simulink model "dSPACE_SIMULINK_MCV_2X"  (Simulink 7.6)
settings: Solver=ode1  StartTime=0.0  StopTime=Inf  FixedStep=(1/10000)  RelTol=1e-3
PostLoadFcn:
  | , if any(exist('dsrtsu_mdlpostloadfcn', 'file') == [2, 3, 6]), try dsrtsu_mdlpostloadfcn('Execute', bdroot); catch fprintf('Error in PostLoadFcn (dsrtsu_mdlpostloadfcn) for model "%s":\n %s\n', bdroot, lasterr); end, end,
values from neighbouring files (symbols this model uses):
  Ap = [0              Cy           0          0 ... (first row only)    [LoadnCheckModel.m]
  Ayaw = [0            Cx        0           0 ... (first row only)    [LoadnCheckModel.m]
  Bp = [0 0 0 KsEL*CwEL/tausEL]'    [LoadnCheckModel.m]
  Byaw = [0     0    0   KsAZ*CwAZ/tausAZ]'    [LoadnCheckModel.m]
  Cp = [1 0 0 0]    [LoadnCheckModel.m]
  Cyaw = [1 0 0 0]    [LoadnCheckModel.m]
  Kpf = KalmanFilter(Ap,Bp,Cp,Dp,Gp,W,V)    [GLTS_2X_master.m]
  Kpmcv = MCVController(Ap,Bp,Cp,Dp,Gp,W,gamma)    [GLTS_2X_master.m]
  Kyf = KalmanFilter(Ayaw, Byaw, Cyaw, Dyaw, Gyaw, W, V)    [GLTS_2X_master.m]
  Kymcv = MCVController(Ayaw,Byaw,Cyaw,Dyaw,Gyaw,W,gamma)    [GLTS_2X_master.m]
libraries: rtilib1104 x2, rti1104serlib x2, simulink x2
settings Model: DSRTSU_INTERNAL_RTI_VER=370  DSRTSU_INTERNAL_RTI_TYPE=rti1104  Creator=Team10  LastModifiedBy=Team10  TunableVars=Aye,Bye,Cye,Dye,Kpf,Kyf,Kyhat,Kylqg  TunableVarsStorageClass=Auto,Auto,Auto,Auto,Auto,Auto,Auto,Auto  TunableVarsTypeQualifier=,,,,,,,  BufferReuse=off
settings DataIOCC: LimitDataPoints=off
settings OptimizationCC: BlockReduction=off  ConditionallyExecuteInputs=off  OptimizeBlockIOStorage=off  BufferReuse=off  ExpressionFolding=off  LocalBlockOutputs=off
settings HardwareCC: ProdIntDivRoundTo=Zero  ProdEndianess=BigEndian  ProdHWDeviceType=Generic->Custom  TargetIntDivRoundTo=Zero  TargetEndianess=BigEndian  TargetHWDeviceType=Generic->Custom
settings RTWCC: SystemTargetFile=rti1104.tlc  MakeCommand=make_rti  TemplateMakefile=rti1104.tmf  Description=dSPACE DS1104 Hardware Platform  ProcessScript=rti1104_make_rtw_hook
settings STFCustomTargetCC: ParMdlRefBuildCompliant=on  GeneratePreprocessorConditionals=Disable all  SystemTargetFile=rti1104.tlc
settings GRTTargetCC: CompOptLevelCompliant=off  MatFileLogging=off  ExtModeMexFile=noextcomm
settings CustomProperty: DataType=RTWOptions_EnumType_C__dSPACE_matlab_rti1104_tlc_rti1104_1InitialSimState  Value=STOP
settings EnumStrPairs: String=RUN

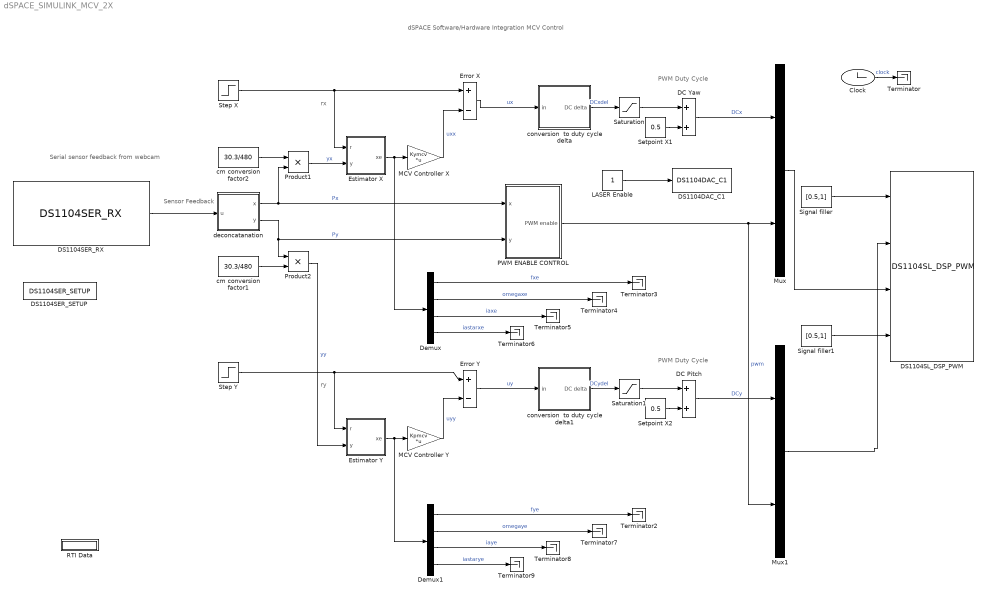
== system dSPACE_SIMULINK_MCV_2X ==
  note: rx
  note: PWM Duty Cycle
  note: dSPACE Software/Hardware Integration MCV Control
  note: Sensor Feedback
  note: Serial sensor feedback from webcam
  note: ry
  note: PWM Duty Cycle
  Clock : Clock
  DC Pitch : Sum
  DC Yaw : Sum
  DS1104DAC_C1 : rtilib1104/DS1104 MASTER PPC/DS1104DAC_C1  SystemSampleTime=-1  ChannelNo=1  InitValue=0  TermMode=0  TermValue=0  Reserved1=[]  Reserved2=[]  Reserved3=[]  Reserved4=[]  DialogFcn=gui1104dac  UnitName={ 'DS1104DAC_C'}  UnitValues={ 1 }  DSProperties=struct('RTI',struct('Version',uint32(1),'BlockType',struct('isSLSource',uint8(0),'isSLSink',uint8(1),'isHWSource',uint8(0),'isHWSink',uint8(1),'isSetup',uint8(0),'isInline',uint8(1),'isNonInline',uint8(0),'isInterrupt',uint8(0),'isChannelwise',uint8(1)),'IOBoardType','DS1104MASTER','UnitType','DAC','Identifier','DAC','DialogType','ML','BlockSet','NONE','SlaveProcessor','NONE'))
  DS1104SER_RX : rti1104serlib/DS1104SER_RX  SystemSampleTime=-1  Reserved1=[]  Reserved2=[]  Reserved3=[]  Reserved4=[]  DSProperties=struct('RTI',struct('IOBoardType',{{'DS1104','SER'}},'SlaveProcessor','NONE','Version',uint32(1),'BlockType',struct('isSLSource',uint8(1),'isSLSink',uint8(1),'isHWSource',uint8(0),'isHWSink',uint8(1),'isSetup',uint8(0),'isInline',uint8(1),'isNonInline',uint8(0),'isInterrupt',uint8(0),'isChannelwise',uint8(1)),'UnitType','GENSER','Identifier','RECEIVE','DialogType','ML','BlockSet','NONE'))  RTIBlockInterface=struct('BlockName',struct('Token',{{'DS1104SER_RX'}}),'InputPortsWidth',int32(1),'InputPortsActive',0,'InputPortsDataType',{{'SS_UINT32'}},'InputPortsName',{{'NumBytes'}},'OutputPortsWidth',int32([8 1 1]),'OutputPortsActive',[1 0 0],'OutputPortsDataType',{{'SS_UINT8','SS_UINT32','SS_INT32'}},'OutputPortsName',{{'RXBytes','NumRXBytes','Status'}},'BlockDisplay',{{['Serial Receive'],'center'}},'IconTransparency','on','ParameterTunableNames',{{}},'InitLevel',2,'DialogFcn','guigenserreceive','MaskDescription',['To read data from the UART SW FIFO.'])  RTIBlockParameters=struct('BoardNo',{{1,'ON',[1 1]}},'ChannelNo',{{1,'ON',[1 1]}},'ChannelNumOf',{{1,'OFF',[]}},'ReceptionDataMode',{{1,'OFF',[]}},'ParamTunableMode',{{2,'OFF',[]}},'BytesRefNumOfT',{{'1','OFF',[1 inf]}},'BytesRefNumOfNT',{{'8','OFF',[1 inf]}},'BytesRefNumOfMax',{{'1','OFF',[1 inf]}},'BytesRefNumOfMode',{{0,'OFF',[]}},'BytesActNumOfMode',{{0,'OFF',[]}},'ReceptionStatusMode',{{0,'OFF',[]}},'FifoSizeDefault',{{64,'OFF',[]}},'TLCFileName',{{'rtigenserreceive','OFF',[]}})  RTISFcnParameters=struct('BoardNo','double','ChannelNo','double','ChannelNumOf','double','ReceptionDataMode','double','ParamTunableMode','double','BytesRefNumOfT','double','BytesRefNumOfNT','double','BytesRefNumOfMax','double','BytesRefNumOfMode','double','BytesActNumOfMode','double','ReceptionStatusMode','double','TLCFileName','char')  RTIBlockParaDefault=struct('BoardNo',1,'ChannelNo',1,'ChannelNumOf',1,'ReceptionDataMode',1,'ParamTunableMode',1,'BytesRefNumOfT',1,'BytesRefNumOfNT',1,'BytesRefNumOfMax',1,'BytesRefNumOfMode',0,'BytesActNumOfMode',1,'ReceptionStatusMode',1,'FifoSizeDefault',64,'TLCFileName','rtigenserreceive')
  DS1104SER_SETUP : rti1104serlib/DS1104SER_SETUP  SystemSampleTime=-1  Reserved1=[]  Reserved2=[]  Reserved3=[]  Reserved4=[]  DSProperties=struct('RTI',struct('IOBoardType',{{'DS1104','SER'}},'SlaveProcessor','NONE','Version',uint32(2),'BlockType',struct('isSLSource',uint8(0),'isSLSink',uint8(0),'isHWSource',uint8(0),'isHWSink',uint8(0),'isSetup',uint8(1),'isInline',uint8(1),'isNonInline',uint8(0),'isInterrupt',uint8(0),'isChannelwise',uint8(1)),'UnitType','GENSER','Identifier','SETUP','DialogType','ML','BlockSet','NONE'))  RTIBlockInterface=struct('BlockName',struct('Token',{{'DS1104SER_SETUP'}}),'BlockDisplay',{{['Serial Setup'],'center'}},'IconTransparency','off','ParameterTunableNames',{{}},'InitLevel',1,'DialogFcn','guigensersetup','MaskDescription',['To set the global specifications for the UART interface.'])  RTIBlockParameters=struct('ParityMode',{{1,'OFF',[1 5]}},'TransceiverMode',{{1,'OFF',[]}},'QuartzFrequency',{{'16000000','OFF',[1 1]}},'BoardNo',{{1,'ON',[1 1]}},'ChannelNo',{{1,'ON',[1 1]}},'ChannelNumOf',{{1,'OFF',[]}},'BaudRate',{{'19200','OFF',[]}},'DataBitsNumOf',{{3,'OFF',[1 4]}},'StopBitsNumOf',{{1,'OFF',[1 3]}},'ReceiveIntLevelUart',{{3,'OFF',[1 4]}},'AutoflowMode',{{1,'OFF',[]}},'FifoSize',{{'64','OFF',[]}},'ReceiveIntLevelFifo',{{0,'OFF',[]}},'FifoOverrunMode',{{2,'OFF',[]}},'FifoBlockSize',{{'8','OFF',[]}},'TermMode',{{1,'OFF',[]}},'TLCFileName',{{'rtigensersetup','OFF',[]}})  RTISFcnParameters=struct('BoardNo','double','ChannelNo','double','ChannelNumOf','double','BaudRate','double','DataBitsNumOf','double','StopBitsNumOf','double','ParityMode','double','TransceiverMode','double','ReceiveIntLevelUart','double','AutoflowMode','double','FifoSize','double','ReceiveIntLevelFifo','double','FifoBlockSize','double','TermMode','double','QuartzFrequency','double','TLCFileName','char')  RTIBlockParaDefault=struct('ParityMode',1,'TransceiverMode',1,'QuartzFrequency',16000000,'BoardNo',1,'ChannelNo',1,'ChannelNumOf',1,'BaudRate',115200,'DataBitsNumOf',4,'StopBitsNumOf',1,'ReceiveIntLevelUart',4,'AutoflowMode',0,'FifoSize',64,'ReceiveIntLevelFifo',0,'FifoOverrunMode',1,'FifoBlockSize',0,'TermMode',1,'TLCFileName','rtigensersetup')
  DS1104SL_DSP_PWM : rtilib1104/DS1104 SLAVE DSP/DS1104SL_DSP_PWM  SystemSampleTime=-1  Parameters=[]  TDef=[]  BoardType=[]  PwmMode=[]  Frequency=[]  InitValue=[]  TermMode=[]  TermValue=[]  Polarity=[]  DialogFcn=[]  Reserved1=[]  Reserved2=[]  Reserved3=[]  Reserved4=[]  Revision=[]  UnitName=[]  UnitValues=[]  DSProperties=struct('RTI',struct('Version',uint32(2),'BlockType',struct('isSLSource',uint8(0),'isSLSink',uint8(1),'isHWSource',uint8(0),'isHWSink',uint8(1),'isSetup',uint8(0),'isInline',uint8(1),'isNonInline',uint8(0),'isInterrupt',uint8(0),'isChannelwise',uint8(0)),'IOBoardType','DS1104SLAVE','UnitType','PWM','Identifier','PWM','DialogType','ML','BlockSet','NONE','SlaveProcessor','F240'))  RTIBlockInterface=struct('InputPortsActive',[1 1 1 1],'InputPortsWidth',int32([2 2 2 2]),'InputPortsName',{{['PWM Channel 1'],['PWM Channel 2'],['PWM Channel 3'],['PWM Channel 4']}},'IWork',{{{'',uint32(4)}}},'DialogFcn','rti1104slavepwmgui','InitLevel',1,'BlockDisplay',{{'','auto'}},'IconTransparency','on','MultiSFcn',4,'BlockName',struct('Token',{{'DS1104SL_DSP_PWM'}}))  RTIBlockParameters=struct('PWMSymmetryMode',{{1,'OFF',[]}},'PWMFrequency',{{'100000','OFF',[]}},'PWMPolarityMode',{{[1 1 1 1 1],'OFF',[]}},'ChannelNo',{{[1 2 3 4],'OFF',[]}},'SuspendModeInit',{{[1 1 1 1 1],'OFF',[]}},'TTLModeInit',{{[2 2 2 2 2],'OFF',[]}},'DutyCycleInitValueCh1',{{'0.5','OFF',[]}},'DutyCycleInitValueCh2',{{'0.5','OFF',[]}},'DutyCycleInitValueCh3',{{'0.5','OFF',[]}},'DutyCycleInitValueCh4',{{'0.5','OFF',[]}},'DutyCycleInitValueCh5',{{'0.5','OFF',[]}},'EnablePWMStop',{{[1 1 1 1 0],'OFF',[]}},'SuspendModeTerm',{{[1 1 1 1 1],'OFF',[]}},'TTLModeTerm',{{[2 2 2 2 2],'OFF',[]}},'DutyCycleTermValueCh1',{{'0.5','OFF',[]}},'DutyCycleTermValueCh2',{{'0.5','OFF',[]}},'DutyCycleTermValueCh3',{{'0.5','OFF',[]}},'DutyCycleTermValueCh4',{{'0.5','OFF',[]}},'DutyCycleTermValueCh5',{{'0.5','OFF',[]}},'TLCFileName',{{'rti1104pwm','OFF',[]}})  RTISFcnParameters=struct('PWMSymmetryMode','double','PWMFrequency','double','PWMPolarityMode','double','ChannelNo','double','SuspendModeInit','double','TTLModeInit','double','DutyCycleInitValueCh1','double','DutyCycleInitValueCh2','double','DutyCycleInitValueCh3','double','DutyCycleInitValueCh4','double','EnablePWMStop','double','SuspendModeTerm','double','TTLModeTerm','double','DutyCycleTermValueCh1','double','DutyCycleTermValueCh2','double','DutyCycleTermValueCh3','double','DutyCycleTermValueCh4','double','TLCFileName','char')  RTIBlockParaDefault=struct('PWMSymmetryMode',1,'PWMFrequency',100,'PWMPolarityMode',[1 1 1 1 1],'ChannelNo',[1 2 3 4],'SuspendModeInit',[1 1 1 1 1],'TTLModeInit',[2 2 2 2 2],'DutyCycleInitValueCh1',0.5,'DutyCycleInitValueCh2',0.5,'DutyCycleInitValueCh3',0.5,'DutyCycleInitValueCh4',0.5,'DutyCycleInitValueCh5',0.5,'EnablePWMStop',[1 1 1 1 0],'SuspendModeTerm',[1 1 1 1 1],'TTLModeTerm',[2 2 2 2 2],'DutyCycleTermValueCh1',0.5,'DutyCycleTermValueCh2',0.5,'DutyCycleTermValueCh3',0.5,'DutyCycleTermValueCh4',0.5,'DutyCycleTermValueCh5',0.5,'TLCFileName','rti1104pwm')
  Demux : Demux
  Demux1 : Demux
  Error X : Sum  Inputs=+-
  Error Y : Sum  Inputs=+-
  Estimator X : Subsystem
  Estimator Y : Subsystem
  LASER Enable : Constant
  MCV Controller X : Gain  Gain=Kymcv  Multiplication=Matrix(K*u)
  MCV Controller Y : Gain  Gain=Kpmcv  Multiplication=Matrix(K*u)
  Mux : Mux  Inputs=2
  Mux1 : Mux  Inputs=2
  PWM ENABLE CONTROL : Subsystem
  Product1 : Product  RndMeth=Zero
  Product2 : Product  RndMeth=Zero
  RTI Data : Subsystem  Tag=struct('RTIDataServer',struct('RTIDataServerVs','2','RTIModelDescription','struct(''main'',''dSPACE_SIMULINK_MCV_2X'',''sub'','''',''isMp'',0)'))  LoadFcn="if exist('rtidc'), try,  rtidc('DataHostBlockClbLoad', gcbh); catch, disp(['Warning: ''LoadFcn'' for RTI Data block failed: ' lasterr]); end, end,"
      settings: CopyFcn="if exist('rtidc'), try,  rtidc('DataHostBlockClbCopy', gcbh); catch, disp(['Warning: ''CopyFcn'' for RTI Data block failed: ' lasterr]); end, end,"  DeleteFcn="if exist('rtidc'), try,  rtidc('DataHostBlockClbDelete', gcbh); catch, disp(['Warning: ''DeleteFcn'' for RTI Data block failed: ' lasterr]); end, end,"  ModelCloseFcn="if exist('rtidc'), try,  rtidc('DataHostBlockClbModelClose', gcbh); catch, disp(['Warning: ''ModelCloseFcn'' for RTI Data block failed: ' lasterr]); end, end,"  PreSaveFcn="if exist('rtidc'), try,  rtidc('DataHostBlockClbPreSave', gcbh); catch, disp(['Warning: ''PreSaveFcn'' for RTI Data block failed: ' lasterr]); end, end,"  PostSaveFcn="if exist('rtidc'), try,  rtidc('DataHostBlockClbPostSave', gcbh); catch, disp(['Warning: ''PostSaveFcn'' for RTI Data block failed: ' lasterr]); end, end,"  NameChangeFcn="if exist('rtidc'), try,  rtidc('DataHostBlockClbNameChange', gcbh); catch, disp(['Warning: ''NameChangeFcn'' for RTI Data block failed: ' lasterr]); end, end,"
      mask Type: RTI_DATA_HOST
      mask Description:
      | RTI Data Block.
      | This block is used by RTI to store internal model-dependent data.
      | Please keep this block on the root level of the model. Deleting this block will result in data loss.
      | 
      | NEVER DELETE OR COPY THIS BLOCK!
      mask Help:
      | RTI Data Block.
      | This block is used by RTI to store internal model-dependent data.
      | Please keep this block on the root level of the model. Deleting this block will result in data loss.
      | 
      | NEVER DELETE OR COPY THIS BLOCK!
      mask Display:
      | text(0.5, 0.5, 'RTI Data', 'HorizontalAlignment', 'center');
      | plot([1 0]);
  Saturation : Saturate
  Saturation1 : Saturate
  Setpoint X1 : Constant  Value=0.5
  Setpoint X2 : Constant  Value=0.5
  Signal filler : Constant  Value=[0.5,1]  VectorParams1D=off
  Signal filler1 : Constant  Value=[0.5,1]  VectorParams1D=off
  Step X : Step  Time=0  After=15.15  SampleTime=0
  Step Y : Step  Time=0  After=15.15  SampleTime=0
  Terminator{,2..9} (9 alike) : Terminator
  cm conversion factor1 : Constant  Value=30.3/480
  cm conversion factor2 : Constant  Value=30.3/480
  conversion  to duty cycle delta : Subsystem
  conversion  to duty cycle delta1 : Subsystem
  deconcatanation : Stateflow chart  TreatAsAtomicUnit=on
  wires:
  deconcatanation/2(y) -> Product2/1, PWM ENABLE CONTROL/2(y)  "Py"
  deconcatanation/1(x) -> Product1/2, PWM ENABLE CONTROL/1(x)  "Px"
  cm conversion factor2/1 -> Product1/1
  cm conversion factor1/1 -> Product2/2
  LASER Enable/1 -> DS1104DAC_C1/1
  Saturation/1 -> DC Yaw/1
  Setpoint X1/1 -> DC Yaw/2
  conversion  to duty cycle delta/1(DC delta) -> Saturation/1  "DCxdel"
  Product1/1 -> Estimator X/2(y)  "yx"
  Error X/1 -> conversion  to duty cycle delta/1(in)  "ux"
  Product2/1 -> Estimator Y/2(y)  "yy"
  MCV Controller X/1 -> Error X/2  "uxx"
  Signal filler/1 -> DS1104SL_DSP_PWM/1
  Signal filler1/1 -> DS1104SL_DSP_PWM/4
  DS1104SER_RX/1 -> deconcatanation/1(u)
  PWM ENABLE CONTROL/1(PWM enable) -> Mux/2, Mux1/2  "pwm"
  DC Yaw/1 -> Mux/1  "DCx"
  Mux/1 -> DS1104SL_DSP_PWM/3
  Mux1/1 -> DS1104SL_DSP_PWM/2
  Demux/1 -> Terminator3/1  "fxe"
  Demux/2 -> Terminator4/1  "omegaxe"
  Demux/3 -> Terminator5/1  "iaxe"
  Demux/4 -> Terminator6/1  "iastarxe"
  Step X/1 -> Error X/1, Estimator X/1(r)
  Estimator X/1(xe) -> MCV Controller X/1, Demux/1
  Clock/1 -> Terminator/1  "clock"
  Saturation1/1 -> DC Pitch/1
  Setpoint X2/1 -> DC Pitch/2
  conversion  to duty cycle delta1/1(DC delta) -> Saturation1/1  "DCydel"
  Error Y/1 -> conversion  to duty cycle delta1/1(in)  "uy"
  MCV Controller Y/1 -> Error Y/2  "uyy"
  DC Pitch/1 -> Mux1/1  "DCy"
  Step Y/1 -> Error Y/1, Estimator Y/1(r)
  Estimator Y/1(xe) -> MCV Controller Y/1, Demux1/1
  Demux1/1 -> Terminator2/1  "fye"
  Demux1/2 -> Terminator7/1  "omegaye"
  Demux1/3 -> Terminator8/1  "iaye"
  Demux1/4 -> Terminator9/1  "iastarye"

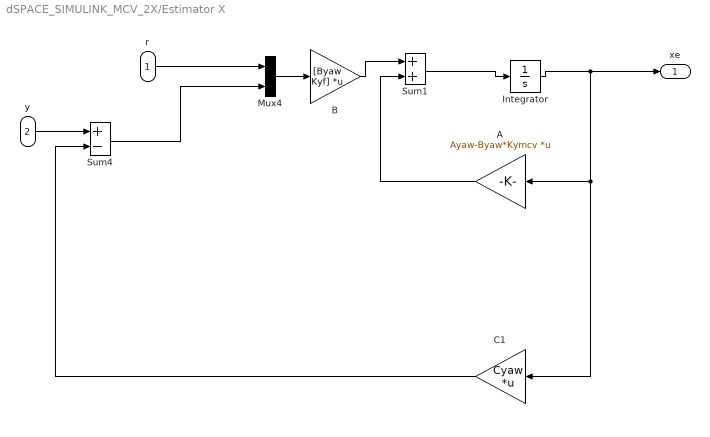
== system dSPACE_SIMULINK_MCV_2X/Estimator X ==
  r : Inport
  y : Inport  Port=2
  A : Gain  Gain=Ayaw-Byaw*Kymcv  Multiplication=Matrix(K*u)
  B : Gain  Gain=[Byaw Kyf]  Multiplication=Matrix(K*u)
  C1 : Gain  Gain=Cyaw  Multiplication=Matrix(K*u)
  Integrator : Integrator  InitialCondition=[0 0 0 0]
  Mux4 : Mux  Inputs=2
  Sum1 : Sum
  Sum4 : Sum  Inputs=+-
  xe : Outport
  wires:
  B/1 -> Sum1/1
  Sum1/1 -> Integrator/1
  Integrator/1 -> A/1, C1/1, xe/1
  r/1 -> Mux4/1
  Mux4/1 -> B/1
  A/1 -> Sum1/2
  y/1 -> Sum4/1
  C1/1 -> Sum4/2
  Sum4/1 -> Mux4/2

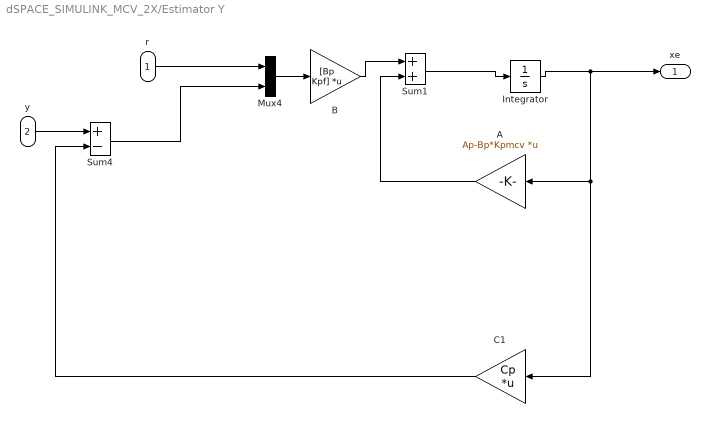
== system dSPACE_SIMULINK_MCV_2X/Estimator Y ==
  r : Inport
  y : Inport  Port=2
  A : Gain  Gain=Ap-Bp*Kpmcv  Multiplication=Matrix(K*u)
  B : Gain  Gain=[Bp Kpf]  Multiplication=Matrix(K*u)
  C1 : Gain  Gain=Cp  Multiplication=Matrix(K*u)
  Integrator : Integrator  InitialCondition=[0 0 0 0]
  Mux4 : Mux  Inputs=2
  Sum1 : Sum
  Sum4 : Sum  Inputs=+-
  xe : Outport
  wires:
  B/1 -> Sum1/1
  Sum1/1 -> Integrator/1
  Integrator/1 -> A/1, C1/1, xe/1
  r/1 -> Mux4/1
  Mux4/1 -> B/1
  A/1 -> Sum1/2
  y/1 -> Sum4/1
  C1/1 -> Sum4/2
  Sum4/1 -> Mux4/2

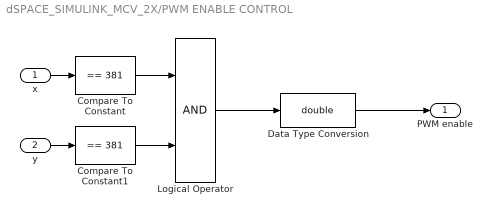
== system dSPACE_SIMULINK_MCV_2X/PWM ENABLE CONTROL ==
  x : Inport
  y : Inport  Port=2
  Compare To Constant : simulink/Logic and Bit Operations/Compare To Constant  SystemSampleTime=-1  relop===  const=381  LogicOutDataTypeMode=boolean
  Compare To Constant1 : simulink/Logic and Bit Operations/Compare To Constant  SystemSampleTime=-1  relop===  const=381  LogicOutDataTypeMode=boolean
  Data Type Conversion : DataTypeConversion  OutDataTypeStr=double
  Logical Operator : Logic  AllPortsSameDT=off  OutDataTypeStr=boolean
  PWM enable : Outport
  wires:
  Compare To Constant/1 -> Logical Operator/1
  Compare To Constant1/1 -> Logical Operator/2
  x/1 -> Compare To Constant/1
  Logical Operator/1 -> Data Type Conversion/1
  y/1 -> Compare To Constant1/1
  Data Type Conversion/1 -> PWM enable/1

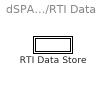
== system dSPACE_SIMULINK_MCV_2X/RTI Data ==
  RTI Data Store : Subsystem  Tag="struct('public',struct('sub',struct('name',{{'dSPACE_SIMULINK_MCV_2X'}},'data',{{struct('TH',struct('thTaskInfo',struct('taskType',{'TIMER','HWINT','TMRINT','SWINT'},'tasksNumOf',{1,0,0,0},'srcIds',{{'TIMERA'},{},{},{}},'taskNames',{{['Timer Task 1']},{},{},{}})),'th_tc',struct('dataType','TASK','taskGroupId','','taskGroupList',{{}},'taskSchedulingPolicy','FCFS','taskType','TIMER','blkh',-1,'srcId','TIMERA','srcSgnName',['Timer A interrupt'],'srcCpuName','','taskName',['Timer Task 1  [0.0001] s'],'taskNameDisplayExt','','smplTime',0.0001,'smplTimeOffs',0,'hasFixedPriority',0,'priority',1,'hasFixedOvc',0,'ovcType',1,'ovcMax',1),'tc_th',struct('dataType','TASK','taskGroupId','','taskGroupList',{{}},'taskSchedulingPolicy','FCFS','taskType','TIMER','blkh',-1,'srcId','TIMERA','srcSgnName',['Timer A interrupt'],'srcCpuName','','taskName',['Timer Task 1  [0.0001] s'],'taskNameDisplayExt','','smplTime',0.0001,'smplTimeOffs',0,'hasFixedPriority',0,'priority',1,'hasFixedOvc',0,'ovcType',1,'ovcMax',1))}})),'private',struct('version',struct('dsVer',uint32(2)),'access',struct('modified',['08-Oct-2013 21:21:43'],'type','Model','isPerm',1)))"
      mask Type: RTI_DATA_STORE
      mask Description:
      | RTI Data Store Block. This block is used by RTI to store internal model dependent data. Deleting this block will result in data loss.
      | 
      | NEVER DELETE, COPY, OR MODIFY THIS BLOCK!
      mask Help:
      | RTI Data Store Block. This block is used by RTI to store internal model dependent data. Deleting this block will result in data loss.
      | 
      | NEVER DELETE, COPY, OR MODIFY THIS BLOCK!
      mask Display: text(0.5, 0.5, ' ', 'HorizontalAlignment', 'center');

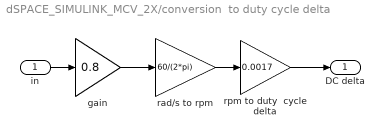
== system dSPACE_SIMULINK_MCV_2X/conversion  to duty cycle delta ==
  in : Inport
  gain : Gain  Gain=0.8
  rad/s to rpm : Gain  Gain=60/(2*pi)
  rpm to duty  cycle delta : Gain  Gain=0.0017
  DC delta : Outport
  wires:
  rad/s to rpm/1 -> rpm to duty  cycle delta/1
  in/1 -> gain/1
  rpm to duty  cycle delta/1 -> DC delta/1
  gain/1 -> rad/s to rpm/1

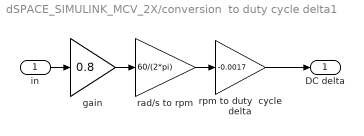
== system dSPACE_SIMULINK_MCV_2X/conversion  to duty cycle delta1 ==
  in : Inport
  gain : Gain  Gain=0.8
  rad/s to rpm : Gain  Gain=60/(2*pi)
  rpm to duty  cycle delta : Gain  Gain=-0.0017
  DC delta : Outport
  wires:
  rad/s to rpm/1 -> rpm to duty  cycle delta/1
  in/1 -> gain/1
  rpm to duty  cycle delta/1 -> DC delta/1
  gain/1 -> rad/s to rpm/1

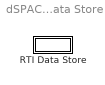
== system dSPACE_SIMULINK_MCV_2X/RTI Data/RTI Data Store ==
  RTI Data Store : Subsystem
      mask Type: RTI_DATA_STORE
      mask Description:
      | RTI Data Store Block. This block is used by RTI to store internal model dependent data. Deleting this block will result in data loss.
      | 
      | NEVER DELETE, COPY, OR MODIFY THIS BLOCK!
      mask Help:
      | RTI Data Store Block. This block is used by RTI to store internal model dependent data. Deleting this block will result in data loss.
      | 
      | NEVER DELETE, COPY, OR MODIFY THIS BLOCK!
      mask Display: text(0.5, 0.5, ' ', 'HorizontalAlignment', 'center');

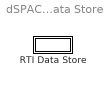
== system dSPACE_SIMULINK_MCV_2X/RTI Data/RTI Data Store/RTI Data Store ==
  RTI Data Store : Subsystem
      mask Type: RTI_DATA_STORE
      mask Description:
      | RTI Data Store Block. This block is used by RTI to store internal model dependent data. Deleting this block will result in data loss.
      | 
      | NEVER DELETE, COPY, OR MODIFY THIS BLOCK!
      mask Help:
      | RTI Data Store Block. This block is used by RTI to store internal model dependent data. Deleting this block will result in data loss.
      | 
      | NEVER DELETE, COPY, OR MODIFY THIS BLOCK!
      mask Display: text(0.5, 0.5, ' ', 'HorizontalAlignment', 'center');

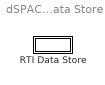
== system dSPACE_SIMULINK_MCV_2X/RTI Data/RTI Data Store/RTI Data Store/RTI Data Store ==
  RTI Data Store : Subsystem
      mask Type: RTI_DATA_STORE
      mask Description:
      | RTI Data Store Block. This block is used by RTI to store internal model dependent data. Deleting this block will result in data loss.
      | 
      | NEVER DELETE, COPY, OR MODIFY THIS BLOCK!
      mask Help:
      | RTI Data Store Block. This block is used by RTI to store internal model dependent data. Deleting this block will result in data loss.
      | 
      | NEVER DELETE, COPY, OR MODIFY THIS BLOCK!
      mask Display: text(0.5, 0.5, ' ', 'HorizontalAlignment', 'center');

== system dSPACE_SIMULINK_MCV_2X/RTI Data/RTI Data Store/RTI Data Store/RTI Data Store/RTI Data Store ==

== matlab function deconcatanation ==
  data: x output double; y output double; u input double
function [x,y] = integ(u)
 
 y = sum(u(1:4));
 x = sum(u(5:8));

    
end
